simulink model "Suspension_nonelinear"  (R2018b)
settings: Solver=VariableStepAuto  StartTime=0.0  StopTime=10.0  RelTol=1e-3
values from neighbouring files (symbols this model uses):
  Ccomp = 600    [CarQuarterParam.m]
  Cext = 1200    [CarQuarterParam.m]
  Ks = 2e4    (= 20000)    [CarQuarterParam.m]
  Ks2 = 20*Ks    (= 400000)    [CarQuarterParam.m]
  x0 = 0.2    [CarQuarterParam.m]
settings Model: Creator=Reece Bell  LastModifiedBy=reece

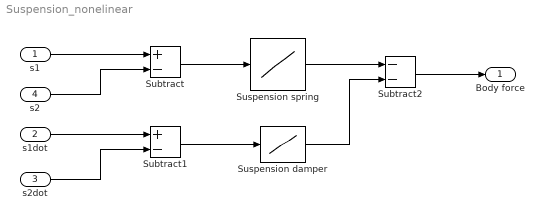
== system Suspension_nonelinear ==
  s1 : Inport
  "s1dot " : Inport  Port=2
  s2dot : Inport  Port=3
  s2 : Inport  Port=4
  Subtract : Sum  Inputs=+-
  Subtract1 : Sum  Inputs=+-
  Subtract2 : Sum  Inputs=--
  Suspension damper : Lookup_n-D  NumberOfTableDimensions=1  BreakpointsForDimension1=[-1,0,1]  Table=[-Ccomp,0,Cext]  InternalRulePriority=Speed  RndMeth=Simplest  InputSameDT=on
  "Suspension spring " : Lookup_n-D  NumberOfTableDimensions=1  BreakpointsForDimension1=[-2*x0, -x0, x0, 2*x0]  Table=[-(Ks + Ks2)*x0, -Ks*x0, Ks*x0, (Ks + Ks2)*x0]  InternalRulePriority=Speed  RndMeth=Simplest  InputSameDT=on
  Body force : Outport
  wires:
  "s1dot "/1 -> Subtract1/1
  Subtract2/1 -> Body force/1
  s2/1 -> Subtract/2
  s2dot/1 -> Subtract1/2
  s1/1 -> Subtract/1
  Subtract/1 -> "Suspension spring "/1
  "Suspension spring "/1 -> Subtract2/1
  Subtract1/1 -> Suspension damper/1
  Suspension damper/1 -> Subtract2/2
